simulink library "Simple_lib"  (R2018b)
settings: Solver=ode45  StartTime=0.0  StopTime=10.0  RelTol=1e-3  EnableMultiTasking=on
undefined symbols (not defined in the file or in its folder): Acceptance, beta, C, C_J, C_P, c_wall, dGain, DiscIntNeverNeededParam, Duplex, Electrical_lib, grab, h_fe, i, i3, K_T, Kman, KmanCE, mu_s, n_rev, R_arm, Simplex, systemTs, tau_0, TinIC, Ts, w_0, wallMass, Watch_lib
libraries: $bdroot x407, PlantUtilityBlockset_lib x30, peGeneralControl x22, simulink x11
(part 6 of 14)

== system Simple_lib/Electrical/BiGain ==
  w : Inport
  Bus Creator1 : BusCreator  Inputs=2
  Bus Selector : BusSelector  OutputSignals=I,C
  Ground : Ground
  Terminator : Terminator
  _in : $bdroot/Rotational/_in  Level=w  Flow=tau
  _out : Subsystem  Tag=Electrical  AncestorBlock=Simple_lib/Electronics/_out  mask{Level=V, Flow=I}
      mask prompts: Level "Level variable name:"; Flow "Flow variable name:"
      mask init:
      | init_out
      mask Display:
      | % This is a new mask on top of the base mask.
      | % Use "View base mask" link below to see the base mask.
      | % Icon for flow out
      | %% Complex icon
      | %plot([0 1 1], [0 0 0.4])
      | %plot([1 1 3], [0.6 1 1])
      | %plot([1 3 2 1 0 2], [0.6 0.6 0.4 0.6 0.4 0.4])
      | %patch([0 2 1],[0.4 0.4 0.6])
      | %plot([3 2 2], [1 1 0.6])
      | %plot([2.2 2.2], [1 0.6])
      | %plot([1.8 1.8], [1 0.6])
      | %plot([1.6 2.4], [0 0])
      | %plot([2 2], [0.1 -0.1])
      | %plot([2 2], [0.4 0.2])
      | %plot([2 2 3], [-0.2 -1 -1])
      | 
      | %color('white')
      | %plot([0 3], [2 2])
      | %plot([0 3], [-2 -2])
      | 
      | %% Bolder icon
      | plot([-1 0 1], [0 -1 0])
      | %patch([-1 1 0 -1], [1 1 2 1]*1-1)
      | patch([-1 -.2 -.2], [0 0 1])
      | patch([1 .2 .2], [0 0 1])
      | %patch( [-0.1 0.1 0.1 -0.1], [0 0 1 1], [1 1 1])
      | plot(0.2*[-1 1],-0.3*[1  1]+0*1.5)
      | plot([0 0],[-0.15 -0.45]+0*1.5)
      | 
      | 
      | color('white')
      | plot( [-1 1], [2 2])
      | plot( [-1 1], -[2 2])
  k_flow1 : Gain  Gain=k_flow
  k_pot : Gain  Gain=k_level
  V : Outport
  wires:
  _out/1(out) -> V/1
  Ground/1 -> Bus Creator1/2  "J"
  Bus Selector/2 -> Terminator/1  "<C>"
  w/1 -> _in/1
  _out/2(backs) -> Bus Selector/1
  k_pot/1 -> _out/1(in)
  Bus Creator1/1 -> _in/2
  k_flow1/1 -> Bus Creator1/1  "tau"
  _in/1 -> k_pot/1
  Bus Selector/1 -> k_flow1/1  "<I>"

== system Simple_lib/Electrical/C ==
  In1 : Inport
  Bus Creator : BusCreator  Inputs=2
  Bus Selector : BusSelector  OutputSignals=V,R
  Constant : Constant  Value=C
  Divide : Product  Inputs=/*
  Ground : Ground
  Ground1 : Ground
  Inflow : $bdroot/Utility/Inflow  SystemSampleTime=-1
  Integrator (Discrete or Continuous) : peGeneralControl/Integrator (Discrete or Continuous)  LabelModeActiveChoice=Discrete  ExternalReset=level  LimitType=Anti-windup  B=inf  A=-inf  Ts=-1
  Outflow : $bdroot/Utility/Outflow  Tag=Electrical  SystemSampleTime=-1
  Sum2 : Sum  Inputs=|+-
  Sum3 : Sum  Inputs=+  CollapseMode=Specified dimension  CollapseDim=2
  Terminator : Terminator
  Weighted Sample Time2 : SampleTimeMath  TsampMathOp=/  weightValue=1
  Out1 : Outport
  wires:
  Outflow/1 -> Out1/1
  Bus Creator/1 -> Outflow/1
  Sum2/1 -> Bus Creator/1  "V"
  Sum3/1 -> Inflow/2, Divide/2  "I"
  Bus Selector/1 -> Sum2/1  "<V>"
  Integrator (Discrete or Continuous)/1 -> Sum2/2
  Outflow/2 -> Sum3/1
  Inflow/1 -> Bus Selector/1
  In1/1 -> Inflow/1
  Bus Selector/2 -> Bus Creator/2, Weighted Sample Time2/1  "<R>"
  Ground/1 -> Integrator (Discrete or Continuous)/3
  Ground1/1 -> Integrator (Discrete or Continuous)/2
  Weighted Sample Time2/1 -> Terminator/1  "1/C"
  Divide/1 -> Integrator (Discrete or Continuous)/1
  Constant/1 -> Divide/1

== system Simple_lib/Electrical/C0 ==
  C : $bdroot/Electrical/C  C=C
      settings: AttributesFormatString=%<C> (F)
  Gnd : $bdroot/Electrical/Gnd  SystemSampleTime=-1
  Out1 : Outport
  wires:
  Gnd/1 -> C/1
  C/1 -> Out1/1

== system Simple_lib/Electrical/C1 ==
  In1 : Inport
  In2 : Inport  Port=2
  1/R1 : Gain  Gain=-1
  1/R2 : Gain  Gain=-1
  Capacitance : Gain  Gain=C
  Discrete-Time Integrator2 : DiscreteIntegrator  gainval=1  SampleTime=Ts  ICPrevOutput=DiscIntNeverNeededParam  ICPrevScaledInput=DiscIntNeverNeededParam
  Simplex : PlantUtilityBlockset_lib/Utility/Push  Tag=Electrical  SystemSampleTime=-1
  Simplex1 : PlantUtilityBlockset_lib/Utility/Push  Tag=Electrical  SystemSampleTime=-1
  Sum : Sum  Inputs=+|+
  Sum1 : Sum  Inputs=|+-
  Unit Delay : UnitDelay  SampleTime=-1
  big : Gain  Gain=100
  wires:
  big/1 -> Discrete-Time Integrator2/1, Capacitance/1
  In1/1 -> Simplex/1
  Simplex/1 -> 1/R2/1
  1/R2/1 -> Sum/1
  Sum/1 -> Sum1/1
  In2/1 -> Simplex1/1
  Simplex1/1 -> Sum/2
  1/R1/1 -> Simplex1/2
  Sum1/1 -> big/1
  Discrete-Time Integrator2/1 -> Sum1/2
  Capacitance/1 -> Unit Delay/1
  Unit Delay/1 -> Simplex/2, 1/R1/1

== system Simple_lib/Electrical/C2 ==
  In1 : Inport
  C1 : $bdroot/Electrical/C1  C=1
  Gnd : $bdroot/Electrical/Gnd  SystemSampleTime=-1
  wires:
  In1/1 -> C1/2
  Gnd/1 -> C1/1

== system Simple_lib/Electrical/Can ==
  note: {\bfCAN - arbitrates contention by {\ithats in ring} algorithm}
      |
      | The bus can arbitrate by broadcasting the minimum contender id and the sum of all contender messages.
      | This mimics the lossless bitwise arbitration method of contention resolution.
  InPot : Inport  Tag=NOFLUX
  FlowSum1 : Sum  Inputs=1  SaturateOnIntegerOverflow=on  InputSameDT=on  OutDataTypeStr=Inherit: Same as first input
  FlowSum2 : Sum  Inputs=3  SaturateOnIntegerOverflow=on  InputSameDT=on  OutDataTypeStr=Inherit: Same as first input
  MinMax : MinMax
  Mux : Mux  Inputs=3
  Mux1 : Mux  Inputs=3
  Mux2 : Mux  Inputs=3
  Selector : Selector  InputPortWidth=3  IndexOptions=Index vector (dialog)  Indices=1  OutputSizes=1
  Selector1 : Selector  InputPortWidth=3  IndexOptions=Index vector (dialog)  Indices=1  OutputSizes=1
  Selector2 : Selector  InputPortWidth=3  IndexOptions=Index vector (dialog)  Indices=1  OutputSizes=1
  Selector3 : Selector  InputPortWidth=3  IndexOptions=Index vector (dialog)  Indices=2  OutputSizes=1
  Selector5 : Selector  InputPortWidth=3  IndexOptions=Index vector (dialog)  Indices=2  OutputSizes=1
  Selector6 : Selector  InputPortWidth=3  IndexOptions=Index vector (dialog)  Indices=2  OutputSizes=1
  Selector7 : Selector  InputPortWidth=3  IndexOptions=Index vector (dialog)  Indices=3  OutputSizes=1
  Selector8 : Selector  InputPortWidth=3  IndexOptions=Index vector (dialog)  Indices=3  OutputSizes=1
  Selector9 : Selector  InputPortWidth=3  IndexOptions=Index vector (dialog)  Indices=3  OutputSizes=1
  OutPot : Outport
  OutFlow : Outport  Tag=NOFLUX  Port=2
  wires:
  InPot/1 -> OutPot/1  "p_DuplexInverter_test0"
  Mux/1 -> MinMax/1
  Mux1/1 -> OutFlow/1
  Selector5/1 -> Mux2/2
  Selector3/1 -> Mux2/1
  Selector6/1 -> Mux2/3
  Mux2/1 -> FlowSum1/1  "msg"
  MinMax/1 -> Mux1/1  "id"
  Selector/1 -> Mux/1
  Selector1/1 -> Mux/2
  Selector2/1 -> Mux/3
  Selector7/1 -> FlowSum2/1
  Selector9/1 -> FlowSum2/3
  Selector8/1 -> FlowSum2/2
  FlowSum2/1 -> Mux1/3
  FlowSum1/1 -> Mux1/2  "msg"

== system Simple_lib/Electrical/Capacitor ==
  In1 : Inport
  Discrete-Time Integrator1 : DiscreteIntegrator  gainval=1  SampleTime=-1  ICPrevOutput=DiscIntNeverNeededParam  ICPrevScaledInput=DiscIntNeverNeededParam
  Gain : Gain  Gain=-1/C
  Input : $bdroot/Utility/Input  Level=V  Flow=I
  Output : $bdroot/Utility/Output  Tag=Electrical  Level=Level  Flow=flow
  Sum : Sum  Inputs=|++
  Sum1 : Sum  Inputs=1
  Out1 : Outport
  wires:
  Discrete-Time Integrator1/1 -> Sum/2
  In1/1 -> Input/1
  Output/1 -> Out1/1
  Output/2 -> Sum1/1
  Input/1 -> Sum/1
  Sum/1 -> Output/1
  Gain/1 -> Discrete-Time Integrator1/1
  Sum1/1 -> Input/2, Gain/1

== system Simple_lib/Electrical/Complex Ammeter ==
  note: $\tau = {L \over R} > \tt{T_s}$
  note: So smaller delay comes from larger resistance
  note: It has to be able to jump through a rate change block!
  + : Inport
  - : Inport  Port=2
  1/R5 : Gain  Gain=-1
  Abs : Abs
  Abs1 : Abs
  Complex to Real-Imag : ComplexToRealImag
  Complex to Real-Imag2 : ComplexToRealImag
  Constant : Constant  Value=Ts
  Constant1 : Constant  Value=1.5
  Discrete-Time Integrator1 : DiscreteIntegrator  gainval=1  SampleTime=Ts  ICPrevOutput=DiscIntNeverNeededParam  ICPrevScaledInput=DiscIntNeverNeededParam
  Divide : Product  Inputs=***
  Divide1 : Product  Inputs=/*
  InNeg : $bdroot/Utility/Input  Level=V  Flow=I
  InPos : $bdroot/Utility/Input  Level=V  Flow=I
  Sum : Sum  Inputs=+|-
  Sum1 : Sum  Inputs=+|+
  Output : Outport
  wires:
  -/1 -> InNeg/1
  +/1 -> InPos/1
  Divide/1 -> Divide1/1  "L"
  Abs/1 -> Sum1/1
  Abs1/1 -> Sum1/2
  Constant/1 -> Divide/2
  Constant1/1 -> Divide/1
  Sum1/1 -> Divide/3
  Complex to Real-Imag/2 -> Abs/1
  Complex to Real-Imag2/2 -> Abs1/1
  Sum/1 -> Divide1/2  "DV"
  Complex to Real-Imag2/1 -> Sum/2
  Complex to Real-Imag/1 -> Sum/1
  1/R5/1 -> InNeg/2
  Discrete-Time Integrator1/1 -> 1/R5/1, Output/1, InPos/2
  InPos/1 -> Complex to Real-Imag/1
  Divide1/1 -> Discrete-Time Integrator1/1
  InNeg/1 -> Complex to Real-Imag2/1

== system Simple_lib/Electrical/Complex Resistance ==
  In1 : Inport
  Constant : Constant  Value=-1
  In : $bdroot/Utility/Input  Tag=Electrical  Level=V  Flow=I
  Out : $bdroot/Utility/Output  Tag=Electrical  Level=Level  Flow=flow
  Real-Imag to Complex : RealImagToComplex
  Sum : Sum  Inputs=|+-
  resistance : Gain  Gain=R
  Out1 : Outport
  wires:
  Out/2 -> In/2, Real-Imag to Complex/1
  Sum/1 -> Out/1
  In/1 -> Sum/1
  Out/1 -> Out1/1
  In1/1 -> In/1
  resistance/1 -> Sum/2
  Constant/1 -> Real-Imag to Complex/2
  Real-Imag to Complex/1 -> resistance/1

== system Simple_lib/Electrical/Controller ==
  InPot : Inport
  InFlow : Inport  Tag=NOFLUX  Port=2
  OutPot : Outport  Tag=NOFLUX
  tag scope: SuggestionTx1Bus_test=global
  wires:
  InPot/1 -> OutPot/1  "pot"
  InFlow/1 -> [SuggestionTx1Bus_test]  "flow"

== system Simple_lib/Electrical/D ==
  note: Put the exponential terms from Ebers Moll in here
  In1 : Inport
  In2 : Inport  Port=2
  1/R1 : Gain  Gain=-1
  1/R2 : Gain  Gain=-1
  Constant : Constant
  Input : $bdroot/Utility/Input  Level=V  Flow=I
  Input1 : $bdroot/Utility/Input  Level=V  Flow=I
  Math Function : Math  SaturateOnIntegerOverflow=on
  Sum : Sum  Inputs=+|+
  Sum1 : Sum  Inputs=|+-
  conductance : Gain  Gain=1/26e-3
  conductance1 : Gain  Gain=1e-12
  wires:
  conductance/1 -> Math Function/1
  In1/1 -> Input/1
  Input/1 -> Sum/1
  Sum/1 -> conductance/1
  In2/1 -> Input1/1
  Input1/1 -> 1/R1/1
  Sum1/1 -> conductance1/1
  conductance1/1 -> Input1/2, 1/R2/1
  Constant/1 -> Sum1/2
  Math Function/1 -> Sum1/1
  1/R2/1 -> Input/2
  1/R1/1 -> Sum/2

== system Simple_lib/Electrical/DC Motor ==
  V_1 : Inport
  V_2 : Inport  Port=2
  Discrete FIR Filter : DiscreteFir  Coefficients=ones(1,10)/10
  Discrete FIR Filter1 : DiscreteFir  Coefficients=ones(1,10)/10
  Divide : Product  Inputs=*/
  Inertia : $bdroot/Rotational/Inertia  I=J_mot
      settings: AttributesFormatString=%<I> kgm^2
  LR : $bdroot/Electronics/LR  L=1e-6  R=R_arm  Phi_0=0
      settings: AttributesFormatString=|
      | %<L> H
      | %<R> Ohm
  Lump : $bdroot/Rotational/Lump  w_0=0  max_accel=inf
      settings: AttributesFormatString=%<w_0> rad/s
  R_Cu : $bdroot/Electronics/R  Commented=on  R=R_arm
      settings: AttributesFormatString=%<R> Ohms
  R_Fe : $bdroot/Electronics/R  R=R_Fe
      settings: AttributesFormatString=%<R> Ohms
  Saturation : Saturate  UpperLimit=1  LowerLimit=0
  Sum : Sum  Inputs=-+|
  Sum2 : Sum  Inputs=|-+
  Terminator1 : Terminator
  Transducer : $bdroot/Electrical/BiGain  k_level=k_flow  k_flow=k_flow
      settings: AttributesFormatString="%<k_flow>   %<k_level>"
  ePower1 : $bdroot/Electrical/Power  SystemSampleTime=-1
  ePower2 : $bdroot/Electrical/Power  SystemSampleTime=-1
  mPower : $bdroot/Rotational/Power  SystemSampleTime=-1
  w : Outport
  wires:
  Divide/1 -> Saturation/1
  Discrete FIR Filter/1 -> Divide/1  "P_mech"
  Discrete FIR Filter1/1 -> Divide/2  "P_elec"
  Saturation/1 -> Terminator1/1  "eta"
  Sum2/1 -> Discrete FIR Filter1/1
  ePower2/2 -> Sum2/1
  V_2/1 -> ePower2/1  "V"
  ePower1/2 -> Sum2/2
  V_1/1 -> ePower1/1  "V_1"
  mPower/2 -> Discrete FIR Filter/1
  mPower/1 -> Transducer/1  "w_load"
  Transducer/1 -> Sum/1  "V"
  Sum/1 -> LR/1
  ePower2/1 -> R_Fe/2, LR/2  "V"
  ePower1/1 -> Sum/2, R_Fe/1
  Lump/1 -> w/1, mPower/1, Inertia/1

== system Simple_lib/Electrical/DI ==
  note: Put the exponential terms from Ebers Moll in here
  note: V_T
  In1 : Inport
  T : Inport  Port=2
  In2 : Inport  Port=3
  1/R1 : Gain  Gain=-1
  Constant : Constant
  Divide : Product  Inputs=*/
  Divide1 : Product  Inputs=**/
  Divide2 : Product  Inputs=*/
  Gain : Gain
  I_S : Gain  Gain=1e-12
  Math Function : Math  SaturateOnIntegerOverflow=on
  Real-Imag to Complex : RealImagToComplex
  Sum : Sum  Inputs=+|-
  Sum1 : Sum  Inputs=-+|
  _1 : $bdroot/Utility/Input  Level=V  Flow=I
  _2 : $bdroot/Utility/Input  Level=V  Flow=I
  k : Constant  Value=1.38e-23
  q : Constant  Value=1.6e-19
  I : Outport
  wires:
  Gain/1 -> Divide2/1
  k/1 -> Divide1/1
  Divide1/1 -> Divide2/2, Divide/2  "V_T"
  q/1 -> Divide1/3
  T/1 -> Divide1/2
  Divide/1 -> Math Function/1
  In1/1 -> _1/1
  _1/1 -> Sum/1
  Sum/1 -> Divide/1  "D_V"
  In2/1 -> _2/1
  Sum1/1 -> I_S/1
  Constant/1 -> Sum1/1
  Math Function/1 -> Sum1/2
  Real-Imag to Complex/1 -> _1/2, 1/R1/1
  _2/1 -> Sum/2
  I_S/1 -> Gain/1, I/1, Real-Imag to Complex/1  "I"
  Divide2/1 -> Real-Imag to Complex/2  "Cond"
  1/R1/1 -> _2/2

== system Simple_lib/Electrical/DV ==
  DV : Inport
  In : Inport  Port=2
  Duplex1 : $bdroot/Utility/Output  Tag=Electrical  Level=Level  Flow=flow
  Input1 : $bdroot/Utility/Input  Level=V  Flow=I
  Input2 : $bdroot/Utility/Input  Level=V  Flow=I
  Sum : Sum  Inputs=++|
  Sum1 : Sum  Inputs=+
  Out : Outport
  wires:
  In/1 -> Input2/1
  Duplex1/1 -> Out/1
  Duplex1/2 -> Sum1/1
  Input2/1 -> Sum/2
  Sum/1 -> Duplex1/1
  DV/1 -> Input1/1
  Sum1/1 -> Input2/2, Input1/2
  Input1/1 -> Sum/1

== system Simple_lib/Electrical/Diode ==
  V1 : Inport
  dV : Inport  Port=2
  V2 : Inport  Port=3
  1/R4 : Gain  Gain=-1
  Discrete-Time Integrator : DiscreteIntegrator  gainval=KmanBE  SampleTime=-1  LimitOutput=on  LowerSaturationLimit=0  ICPrevOutput=DiscIntNeverNeededParam  ICPrevScaledInput=DiscIntNeverNeededParam
  Input : $bdroot/Utility/Input  Level=V  Flow=I
  Input1 : $bdroot/Utility/Input  Level=V  Flow=I
  Sum : Sum  Inputs=++-
  I_12 : Outport
  wires:
  1/R4/1 -> Input1/2
  dV/1 -> Sum/2
  Input1/1 -> Sum/3
  Discrete-Time Integrator/1 -> 1/R4/1, I_12/1, Input/2
  V2/1 -> Input1/1
  Sum/1 -> Discrete-Time Integrator/1
  Input/1 -> Sum/1
  V1/1 -> Input/1

== system Simple_lib/Electrical/E1 ==
  In1 : Inport
  Bus Creator : BusCreator  Inputs=2
  Ground1 : Ground
  Out1 : Outport
  wires:
  In1/1 -> Bus Creator/1  "V"
  Ground1/1 -> Bus Creator/2  "R"
  Bus Creator/1 -> Out1/1

== system Simple_lib/Electrical/EMF ==
  In1 : Inport
  Constant : Constant  Value=Vbatt
  Input1 : $bdroot/Utility/Input  Level=V  Flow=I
  Sum : Sum  Inputs=|++
  Sum1 : Sum  Inputs=+
  _ : $bdroot/Utility/Output  Tag=Electrical  Level=Level  Flow=flow
  Out1 : Outport
  wires:
  _/1 -> Out1/1
  Input1/1 -> Sum/1
  _/2 -> Sum1/1
  Constant/1 -> Sum/2
  Sum/1 -> _/1
  In1/1 -> Input1/1
  Sum1/1 -> Input1/2

== system Simple_lib/Electrical/EMachine  ==
  note: Torque Constant = 60/2/pi/K_V
  K : Inport
  V_in : Inport  Port=2
  w_rot : Inport  Port=3
  w_stat : Inport  Port=4
  Gain : Gain  Gain=-1
  Input : $bdroot/Utility/Input  Level=V  Flow=I
  Input1 : $bdroot/Utility/Input  Level=V  Flow=I
  Input2 : $bdroot/Utility/Input  Level=V  Flow=I
  Output : $bdroot/Utility/Output  Tag=Electrical  Level=Level  Flow=flow
  Sum : Sum  Inputs=-+|
  Sum1 : Sum  Inputs=|+-
  Sum3 : Sum  Inputs=+
  Times : Product  Inputs=**
  Times2 : Product  Inputs=**
  V_out : Outport
  wires:
  Gain/1 -> Input1/2
  Times2/1 -> Input2/2, Gain/1
  Times/1 -> Sum/1
  Sum3/1 -> Times2/2, Input/2
  Input2/1 -> Sum1/1
  Input1/1 -> Sum1/2
  w_stat/1 -> Input1/1
  Sum1/1 -> Times/2
  K/1 -> Times/1, Times2/1
  Output/2 -> Sum3/1
  Output/1 -> V_out/1
  Input/1 -> Sum/2
  w_rot/1 -> Input2/1
  V_in/1 -> Input/1
  Sum/1 -> Output/1

== system Simple_lib/Electrical/Flow ==
  In1 : Inport
  1/R1 : Gain  Gain=-1
  Flow : Scope
      settings: Tag=I
  Input2 : $bdroot/Utility/Input  Level=V  Flow=I
  _ : $bdroot/Utility/Output  Tag=Electrical  Level=Level  Flow=flow
  Out1 : Outport
  wires:
  Input2/1 -> _/1
  _/2 -> Input2/2, 1/R1/1
  In1/1 -> Input2/1
  _/1 -> Out1/1
  1/R1/1 -> Flow/1

== system Simple_lib/Electrical/Forward ==
  In1 : Inport
  Discrete-Time Integrator1 : DiscreteIntegrator  gainval=1/0.01  InitialCondition=-deltaV  SampleTime=Ts  LimitOutput=on  LowerSaturationLimit=-deltaV  ICPrevOutput=DiscIntNeverNeededParam  ICPrevScaledInput=DiscIntNeverNeededParam
  Input : $bdroot/Utility/Input  Level=V  Flow=I
  Sum : Sum  Inputs=|++
  _ : $bdroot/Utility/Output  Tag=Electrical  Level=Level  Flow=flow
  Out1 : Outport
  wires:
  Discrete-Time Integrator1/1 -> Sum/2
  _/1 -> Out1/1
  Sum/1 -> _/1
  _/2 -> Discrete-Time Integrator1/1, Input/2
  Input/1 -> Sum/1
  In1/1 -> Input/1

== system Simple_lib/Electrical/Gnd ==
  Input : Inport
  Bus Creator1 : BusCreator  Inputs=2
  Ground2 : Ground
  Ground3 : Ground
  I1 : $bdroot/Electrical/I1  SystemSampleTime=-1
  Output : Outport
  wires:
  Ground2/1 -> Bus Creator1/2  "R"
  Input/1 -> I1/1
  Ground3/1 -> Bus Creator1/1  "V"
  Bus Creator1/1 -> I1/2
  I1/1 -> Output/1  "I1"

== system Simple_lib/Electrical/Grnd ==
  Constant : Constant  Value=0
  Sum : Sum  Inputs=+
  _ : $bdroot/Utility/Output  Tag=Electrical  Level=Level  Flow=flow
  Gnd : Outport
  i : Outport  Port=2
  wires:
  _/1 -> Gnd/1
  Constant/1 -> _/1
  _/2 -> Sum/1
  Sum/1 -> i/1

== system Simple_lib/Electrical/H ==
  + : Inport
  Sw : Inport  Port=2
  - : Inport  Port=3
  Input1 : $bdroot/Utility/Input  Level=V  Flow=I
  Input2 : $bdroot/Utility/Input  Level=V  Flow=I
  Multiply : Product
  Multiply1 : Product
  Sum1 : Sum  Inputs=+
  Sum2 : Sum  Inputs=+
  Switch Volts : Subsystem
  _ : $bdroot/Utility/Output  Tag=Electrical  Level=Level  Flow=flow
  _1 : $bdroot/Utility/Output  Tag=Electrical  Level=Level  Flow=flow
  u : Outport
  v : Outport  Port=2
  wires:
  Sum1/1 -> Multiply/1
  Sum2/1 -> Multiply1/2
  Switch Volts/1(uSw) -> _/1
  Switch Volts/2(vSw) -> _1/1
  Multiply1/1 -> Input2/2
  Multiply/1 -> Input1/2
  Sw/1 -> Switch Volts/2(Sw), Multiply/2, Multiply1/1
  Input1/1 -> Switch Volts/1(u)
  +/1 -> Input1/1
  _1/2 -> Sum2/1
  _/2 -> Sum1/1
  _/1 -> u/1
  _1/1 -> v/1
  Input2/1 -> Switch Volts/3(v)
  -/1 -> Input2/1

== system Simple_lib/Electrical/H Bridge ==
  + : Inport
  ctrl : Inport  Port=2
  - : Inport  Port=3
  1-D Lookup Table1 : Lookup_n-D  NumberOfTableDimensions=1  BreakpointsForDimension1=[-1 0 1]  Table=[1 0 0]  InterpMethod=Nearest  InternalRulePriority=Speed  RndMeth=Simplest  InputSameDT=on
  1-D Lookup Table2 : Lookup_n-D  NumberOfTableDimensions=1  BreakpointsForDimension1=[-1 0 1]  Table=[0 0 1]  InterpMethod=Nearest  InternalRulePriority=Speed  RndMeth=Simplest  InputSameDT=on
  1-D Lookup Table3 : Lookup_n-D  NumberOfTableDimensions=1  BreakpointsForDimension1=[-1 0 1]  Table=[1 0 0]  InterpMethod=Nearest  InternalRulePriority=Speed  RndMeth=Simplest  InputSameDT=on
  1-D Lookup Table4 : Lookup_n-D  NumberOfTableDimensions=1  BreakpointsForDimension1=[-1 0 1]  Table=[0 0 1]  InterpMethod=Nearest  InternalRulePriority=Speed  RndMeth=Simplest  InputSameDT=on
  EMF1 : $bdroot/Electrical/EMF  Vbatt=4
  EMF2 : $bdroot/Electrical/EMF  Vbatt=4
  Tran{,1..3} (4 alike) : $bdroot/Electrical/Tran  SystemSampleTime=-1
  u : Outport
  v : Outport  Port=2
  wires:
  1-D Lookup Table3/1 -> Tran2/1
  1-D Lookup Table1/1 -> Tran1/1
  1-D Lookup Table2/1 -> Tran/1
  1-D Lookup Table4/1 -> Tran3/1
  ctrl/1 -> 1-D Lookup Table1/1, 1-D Lookup Table4/1, 1-D Lookup Table2/1, 1-D Lookup Table3/1
  EMF1/1 -> v/1
  -/1 -> Tran1/2, Tran3/2
  +/1 -> Tran/2, Tran2/2
  Tran3/1 -> ?
  Tran2/1 -> EMF1/1
  EMF2/1 -> u/1
  Tran/1 -> EMF2/1
  Tran1/1 -> ?

== system Simple_lib/Electrical/I1 ==
  note: $\tau = {L \over R} > \tt{T_s}$
  note: So smaller delay comes from larger resistance
  In1 : Inport
  In2 : Inport  Port=2
  Bus Selector : BusSelector  OutputSignals=V,R
  Bus Selector1 : BusSelector  OutputSignals=R,V
  Divide : Product  Inputs=/*
  Gain : Gain  Gain=-1
  Ground : Ground
  Ground1 : Ground
  Inflow1 : $bdroot/Utility/Inflow  SystemSampleTime=-1
  Inflow2 : $bdroot/Utility/Inflow  SystemSampleTime=-1
  Integrator (Discrete or Continuous) : peGeneralControl/Integrator (Discrete or Continuous)  LabelModeActiveChoice=Discrete  ExternalReset=level  LimitType=Anti-windup  B=inf  A=-inf  Ts=-1
  Sum : Sum  Inputs=+|-
  Sum1 : Sum  Inputs=+|+
  Weighted Sample Time2 : SampleTimeMath  TsampMathOp=*  weightValue=1
  I : Outport
  wires:
  Sum1/1 -> Weighted Sample Time2/1
  Divide/1 -> Integrator (Discrete or Continuous)/1
  In2/1 -> Inflow2/1
  In1/1 -> Inflow1/1
  Sum/1 -> Divide/2
  Integrator (Discrete or Continuous)/1 -> Gain/1, I/1, Inflow1/2
  Inflow2/1 -> Bus Selector1/1
  Weighted Sample Time2/1 -> Divide/1  "L"
  Gain/1 -> Inflow2/2
  Bus Selector/2 -> Sum1/1  "<R>"
  Bus Selector/1 -> Sum/1  "<V>"
  Ground/1 -> Integrator (Discrete or Continuous)/3
  Bus Selector1/2 -> Sum/2  "<V>"
  Ground1/1 -> Integrator (Discrete or Continuous)/2
  Bus Selector1/1 -> Sum1/2  "<R>"
  Inflow1/1 -> Bus Selector/1

== system Simple_lib/Electrical/I_1 ==
  In1 : Inport
  In2 : Inport  Port=2
  Bus Selector : BusSelector  OutputSignals=V,R
  Bus Selector1 : BusSelector  OutputSignals=R,V
  Divide : Product  Inputs=/*
  Gain : Gain  Gain=-1
  Ground : Ground
  Ground1 : Ground
  Inflow1 : $bdroot/Utility/Inflow  SystemSampleTime=-1
  Inflow2 : $bdroot/Utility/Inflow  SystemSampleTime=-1
  Integrator (Discrete or Continuous) : peGeneralControl/Integrator (Discrete or Continuous)  LabelModeActiveChoice=Discrete  ExternalReset=level  LimitType=Anti-windup  B=inf  A=-inf  Ts=-1
  Sum : Sum  Inputs=+|-
  Sum1 : Sum  Inputs=+|+
  Weighted Sample Time2 : SampleTimeMath  TsampMathOp=*  weightValue=1
  I : Outport
  wires:
  Inflow1/1 -> Bus Selector/1
  Inflow2/1 -> Bus Selector1/1
  Sum/1 -> Divide/2
  Integrator (Discrete or Continuous)/1 -> Gain/1, I/1, Inflow1/2
  In1/1 -> Inflow1/1
  In2/1 -> Inflow2/1
  Ground/1 -> Integrator (Discrete or Continuous)/3
  Ground1/1 -> Integrator (Discrete or Continuous)/2
  Bus Selector/1 -> Sum/1  "<V>"
  Bus Selector1/2 -> Sum/2  "<V>"
  Bus Selector1/1 -> Sum1/2  "<R>"
  Bus Selector/2 -> Sum1/1  "<R>"
  Weighted Sample Time2/1 -> Divide/1  "L"
  Gain/1 -> Inflow2/2
  Divide/1 -> Integrator (Discrete or Continuous)/1
  Sum1/1 -> Weighted Sample Time2/1

== system Simple_lib/Electrical/I_src ==
  In1 : Inport
  In3 : Inport  Port=2
  1/R1 : Gain  Gain=-1
  1/R2 : Gain  Gain=-1
  Duplex1 : $bdroot/Utility/Output  Tag=Electrical  Level=Level  Flow=flow
  Input : $bdroot/Utility/Input  Level=V  Flow=I
  Input1 : $bdroot/Utility/Input  Level=V  Flow=I
  Sum : Sum  Inputs=+|+
  Out1 : Outport
  wires:
  1/R2/1 -> Sum/1
  1/R1/1 -> Input/2
  In1/1 -> Input/1
  Input/1 -> 1/R2/1
  Duplex1/1 -> Out1/1
  In3/1 -> Input1/1
  Input1/1 -> Sum/2
  Duplex1/2 -> 1/R1/1, Input1/2
  Sum/1 -> Duplex1/1

== system Simple_lib/Electrical/Inline Ammeter ==
  In1 : Inport
  Input2 : $bdroot/Utility/Input  Level=V  Flow=I
  Sum : Sum  Inputs=+
  _ : $bdroot/Utility/Output  Tag=Electrical  Level=Level  Flow=flow
  Out1 : Outport
  Out2 : Outport  Port=2
  wires:
  Sum/1 -> Out2/1
  In1/1 -> Input2/1
  _/1 -> Out1/1
  Input2/1 -> _/1
  _/2 -> Input2/2, Sum/1

== system Simple_lib/Electrical/Isrc ==
  In1 : Inport
  In2 : Inport  Port=2
  In3 : Inport  Port=3
  1/R1 : Gain  Gain=-1
  1/R2 : Gain  Gain=-1
  Input : $bdroot/Utility/Input  Level=V  Flow=I
  Input1 : $bdroot/Utility/Input  Level=V  Flow=I
  Sum : Sum  Inputs=+|+
  Out1 : Outport
  wires:
  In2/1 -> 1/R1/1, Input1/2
  Input1/1 -> Sum/2
  In3/1 -> Input1/1
  Sum/1 -> Out1/1
  Input/1 -> 1/R2/1
  In1/1 -> Input/1
  1/R1/1 -> Input/2
  1/R2/1 -> Sum/1

== system Simple_lib/Electrical/L ==
  In1 : Inport
  In2 : Inport  Port=2
  1/R2 : Gain  Gain=-1
  1/R3 : Gain  Gain=1/L
  1/R5 : Gain  Gain=-1
  Discrete-Time Integrator1 : DiscreteIntegrator  gainval=1  SampleTime=Ts  ICPrevOutput=DiscIntNeverNeededParam  ICPrevScaledInput=DiscIntNeverNeededParam
  Input : $bdroot/Utility/Input  Level=V  Flow=I
  Input1 : $bdroot/Utility/Input  Level=V  Flow=I
  Sum : Sum  Inputs=+|+
  i12 : Outport
  wires:
  1/R3/1 -> Input1/2, 1/R5/1
  Input1/1 -> Sum/2
  In2/1 -> Input1/1
  Sum/1 -> Discrete-Time Integrator1/1
  1/R2/1 -> Sum/1
  Input/1 -> 1/R2/1
  In1/1 -> Input/1
  Discrete-Time Integrator1/1 -> 1/R3/1
  1/R5/1 -> i12/1, Input/2

== system Simple_lib/Electrical/L_ ==
  note: $\Phi \text{ is in Weber = Volt seconds} }$
  V_in : Inport
  Phi_in : Inport  Port=2
  Derivative : Derivative
  Duplex : $bdroot/Utility/Output  Tag=Electrical  Level=Level  Flow=flow
  Inductance per turn : Gain  Gain=L_turn
  Simplex : $bdroot/Utility/Input  Tag=Electrical  Level=V  Flow=I
  Sum : Sum  Inputs=|++
  Sum1 : Sum  Inputs=++|
  Turns : Gain  Gain=N
  V_out : Outport
  Phi_out : Outport  Port=2
  wires:
  Sum/1 -> Duplex/1
  Simplex/1 -> Sum/1
  Duplex/1 -> V_out/1
  V_in/1 -> Simplex/1
  Inductance per turn/1 -> Sum1/2, Phi_out/1
  Duplex/2 -> Simplex/2, Inductance per turn/1
  Derivative/1 -> Sum/2
  Phi_in/1 -> Sum1/1
  Sum1/1 -> Turns/1
  Turns/1 -> Derivative/1

== system Simple_lib/Electrical/L__ ==
  note: $\Phi \text{ is in Weber = Volt seconds} }$
  V_in : Inport
  Derivative : Derivative
  Duplex : $bdroot/Utility/Output  Tag=Electrical  Level=Level  Flow=flow
  Inductance : Gain  Gain=L
  Simplex : $bdroot/Utility/Input  Tag=Electrical  Level=V  Flow=I
  Sum : Sum  Inputs=|++
  V_out : Outport
  wires:
  Inductance/1 -> Derivative/1
  Derivative/1 -> Sum/2
  Duplex/2 -> Simplex/2, Inductance/1
  V_in/1 -> Simplex/1
  Duplex/1 -> V_out/1
  Simplex/1 -> Sum/1
  Sum/1 -> Duplex/1

== system Simple_lib/Electrical/L_thru ==
  In1 : Inport
  Discrete-Time Integrator1 : DiscreteIntegrator  gainval=1  SampleTime=Ts  ICPrevOutput=DiscIntNeverNeededParam  ICPrevScaledInput=DiscIntNeverNeededParam
  Duplex : $bdroot/Utility/Output  Tag=Electrical  Level=Level  Flow=flow
  Inductance : Gain  Gain=L
  Simplex : $bdroot/Utility/Input  Tag=Electrical  Level=V  Flow=I
  Sum : Sum  Inputs=|++
  Sum1 : Sum  Inputs=|+-
  big : Gain  Gain=100
  Out1 : Outport
  wires:
  Sum/1 -> Duplex/1
  Sum1/1 -> big/1
  Simplex/1 -> Sum/1
  Duplex/2 -> Simplex/2, Sum1/1
  Duplex/1 -> Out1/1
  In1/1 -> Simplex/1
  big/1 -> Discrete-Time Integrator1/1, Inductance/1
  Discrete-Time Integrator1/1 -> Sum1/2
  Inductance/1 -> Sum/2

== system Simple_lib/Electrical/Li ==
  In1 : Inport
  In2 : Inport  Port=2
  1/R2 : Gain  Gain=-1
  1/R3 : Gain  Gain=1/L
  1/R5 : Gain  Gain=-1
  Constant : Constant  Value=i/1000
  Discrete-Time Integrator1 : DiscreteIntegrator  gainval=1  SampleTime=Ts  ICPrevOutput=DiscIntNeverNeededParam  ICPrevScaledInput=DiscIntNeverNeededParam
  Input : $bdroot/Utility/Input  Level=V  Flow=I
  Input1 : $bdroot/Utility/Input  Level=V  Flow=I
  Sum : Sum  Inputs=+|+
  Sum1 : Sum  Inputs=++|
  wires:
  1/R3/1 -> Input1/2, 1/R5/1
  Input1/1 -> Sum/2
  In2/1 -> Input1/1
  Sum/1 -> Discrete-Time Integrator1/1
  1/R2/1 -> Sum/1
  Input/1 -> 1/R2/1
  In1/1 -> Input/1
  Discrete-Time Integrator1/1 -> Sum1/2
  1/R5/1 -> Input/2
  Sum1/1 -> 1/R3/1
  Constant/1 -> Sum1/1

== system Simple_lib/Electrical/Li1 ==
  note: So smaller delay comes from larger resistance
  note: $\tau = {L \over R} > \tt{T_s}$
  In1 : Inport
  In2 : Inport  Port=2
  1/R5 : Gain  Gain=-1
  Abs : Abs
  Abs1 : Abs
  Complex to Real-Imag : ComplexToRealImag
  Complex to Real-Imag2 : ComplexToRealImag
  Constant : Constant  Value=Ts
  Constant1 : Constant  Value=1.01
  Discrete-Time Integrator1 : DiscreteIntegrator  gainval=1  SampleTime=Ts  ICPrevOutput=DiscIntNeverNeededParam  ICPrevScaledInput=DiscIntNeverNeededParam
  Divide : Product  Inputs=///*
  Input : $bdroot/Utility/Input  Level=V  Flow=I
  Input1 : $bdroot/Utility/Input  Level=V  Flow=I
  Max : MinMax  Function=max  Inputs=2
  Sum : Sum  Inputs=+|-
  Output : Outport
  wires:
  Input1/1 -> Complex to Real-Imag2/1
  In2/1 -> Input1/1
  Divide/1 -> Discrete-Time Integrator1/1
  Input/1 -> Complex to Real-Imag/1
  Discrete-Time Integrator1/1 -> 1/R5/1, Output/1, Input/2
  1/R5/1 -> Input1/2
  In1/1 -> Input/1
  Complex to Real-Imag/1 -> Sum/1
  Complex to Real-Imag2/1 -> Sum/2
  Sum/1 -> Divide/4
  Complex to Real-Imag2/2 -> Abs1/1
  Complex to Real-Imag/2 -> Abs/1
  Max/1 -> Divide/3
  Constant1/1 -> Divide/1
  Constant/1 -> Divide/2
  Abs1/1 -> Max/2
  Abs/1 -> Max/1

== system Simple_lib/Electrical/Magnetic Field ==
  In1 : Inport
  Duplex : $bdroot/Utility/Output  Tag=Electrical  Level=Level  Flow=flow
  Simplex : $bdroot/Utility/Input  Tag=Electrical  Level=V  Flow=I
  Sum1 : Sum  Inputs=+
  k_flow : Gain  Gain=k_flo
  k_pot : Gain  Gain=k_lev
  Out1 : Outport
  wires:
  Sum1/1 -> k_flow/1
  k_pot/1 -> Duplex/1
  k_flow/1 -> Simplex/2
  In1/1 -> Simplex/1
  Simplex/1 -> k_pot/1
  Duplex/1 -> Out1/1
  Duplex/2 -> Sum1/1

== system Simple_lib/Electrical/Meter ==
  In1 : Inport
  Complex to Real-Imag : ComplexToRealImag
  Input2 : $bdroot/Utility/Input  Level=V  Flow=I
  Sum : Sum  Inputs=+
  Terminator : Terminator
  _ : $bdroot/Utility/Output  Tag=Electrical  Level=Level  Flow=flow
  Out1 : Outport
  Out2 : Outport  Port=2
  wires:
  Sum/1 -> Complex to Real-Imag/1
  In1/1 -> Input2/1
  _/1 -> Out1/1
  _/2 -> Sum/1, Input2/2
  Input2/1 -> _/1
  Complex to Real-Imag/1 -> Out2/1
  Complex to Real-Imag/2 -> Terminator/1

== system Simple_lib/Electrical/NPN ==
  Collector : Inport
  Base : Inport  Port=2
  Emitter : Inport  Port=3
  DiodeBE : $bdroot/Electrical/SimpleDiode  K_diode=KmanBE
  DiodeCE : $bdroot/Electrical/SimpleDiode  K_diode=KmanCE
  Transistor Action : Subsystem
  wires:
  Transistor Action/1(dV_BE) -> DiodeBE/2
  Transistor Action/2(dV_CE) -> DiodeCE/2
  Collector/1 -> DiodeCE/1
  Base/1 -> DiodeBE/1
  Emitter/1 -> DiodeBE/3, DiodeCE/3

== system Simple_lib/Electrical/NPNwp ==
  Collector : Inport
  Base : Inport  Port=2
  Emitter : Inport  Port=3
  Constant : Constant  Value=-0.7
  Constant1 : Constant  Value=-0.7
  Diode : $bdroot/Electrical/Diode  SystemSampleTime=-1
  Diode1 : $bdroot/Electrical/Diode  SystemSampleTime=-1
  Isrc : $bdroot/Electrical/Isrc  SystemSampleTime=-1
  Isrc1 : $bdroot/Electrical/Isrc  SystemSampleTime=-1
  Sum : Sum  Inputs=+|-
  Terminator : Terminator
  Terminator1 : Terminator
  alpha_F : Gain  Gain=-0.98
  alpha_R : Gain  Gain=0.9
  Ic : Outport
  wires:
  Isrc/1 -> Terminator1/1
  Isrc1/1 -> Terminator/1
  Emitter/1 -> Diode1/3, Isrc1/1
  Base/1 -> Diode1/1, Diode/1, Isrc1/3, Isrc/3
  Collector/1 -> Diode/3, Isrc/1
  Diode/1 -> [I_CD], Sum/2
  [I_ED] -> alpha_F/1
  alpha_F/1 -> Sum/1, Isrc/2
  [I_CD] -> alpha_R/1
  alpha_R/1 -> Isrc1/2
  Diode1/1 -> [I_ED]
  Constant/1 -> Diode/2
  Constant1/1 -> Diode1/2
  Sum/1 -> Ic/1

== system Simple_lib/Electrical/OpAmp ==
  + : Inport
  - : Inport  Port=2
  Discrete-Time Integrator : DiscreteIntegrator  gainval=K_op  SampleTime=-1  ICPrevOutput=DiscIntNeverNeededParam  ICPrevScaledInput=DiscIntNeverNeededParam
  Sum : Sum  Inputs=+|-
  Out1 : Outport
  wires:
  +/1 -> Sum/1
  Sum/1 -> Discrete-Time Integrator/1
  -/1 -> Sum/2
  Discrete-Time Integrator/1 -> Out1/1

== system Simple_lib/Electrical/P ==
  Discrete-Time Integrator1 : DiscreteIntegrator  gainval=1  SampleTime=Ts  ICPrevOutput=DiscIntNeverNeededParam  ICPrevScaledInput=DiscIntNeverNeededParam
  Gain : Gain  Gain=-1/C_P
  Sum1 : Sum  Inputs=1
  _ : $bdroot/Utility/Output  Tag=Electrical  Level=Level  Flow=flow
  Out1 : Outport
  wires:
  _/1 -> Out1/1
  _/2 -> Sum1/1
  Discrete-Time Integrator1/1 -> Gain/1
  Sum1/1 -> Discrete-Time Integrator1/1
  Gain/1 -> _/1

== system Simple_lib/Electrical/PNPwp ==
  Collector : Inport
  Base : Inport  Port=2
  Emitter : Inport  Port=3
  Constant : Constant  Value=-0.7
  Constant1 : Constant  Value=-0.7
  Diode : $bdroot/Electrical/Diode  SystemSampleTime=-1
  Diode1 : $bdroot/Electrical/Diode  SystemSampleTime=-1
  Isrc : $bdroot/Electrical/Isrc  SystemSampleTime=-1
  Isrc1 : $bdroot/Electrical/Isrc  SystemSampleTime=-1
  Sum : Sum  Inputs=-|+
  Terminator : Terminator
  Terminator1 : Terminator
  alpha_F : Gain  Gain=-0.98
  alpha_R : Gain  Gain=0.9
  Ic : Outport
  wires:
  Base/1 -> Diode/3, Diode1/3, Isrc/1, Isrc1/1
  Isrc1/1 -> Terminator1/1
  Isrc/1 -> Terminator/1
  Emitter/1 -> Diode/1, Isrc/3
  Collector/1 -> Diode1/1, Isrc1/3
  Diode1/1 -> Sum/2, [I_CD]
  [I_ED] -> alpha_F/1
  alpha_F/1 -> Sum/1, Isrc1/2
  [I_CD] -> alpha_R/1
  alpha_R/1 -> Isrc/2
  Diode/1 -> [I_ED]
  Constant/1 -> Diode1/2
  Constant1/1 -> Diode/2
  Sum/1 -> Ic/1

== system Simple_lib/Electrical/Pi ==
  note: RC ~= Ts
      | so want C to just exceed Ts * the max conductance
  Abs : Abs
  Complex to Real-Imag : ComplexToRealImag
  Constant : Constant  Value=-Ts
  Constant1 : Constant  Value=2
  Discrete-Time Integrator1 : DiscreteIntegrator  gainval=1  SampleTime=Ts  ICPrevOutput=DiscIntNeverNeededParam  ICPrevScaledInput=DiscIntNeverNeededParam
  Display : Display
  Divide : Product  Inputs=***
  Divide1 : Product  Inputs=*/
  Min : MinMax  Function=max
  Scope : Scope
  Sum1 : Sum  Inputs=1
  _ : $bdroot/Utility/Output  Tag=Electrical  Level=Level  Flow=flow
  Out1 : Outport
  wires:
  Complex to Real-Imag/2 -> Abs/1
  Divide/1 -> Divide1/2, Display/1
  Min/1 -> Divide/1
  _/1 -> Out1/1
  _/2 -> Complex to Real-Imag/1
  Discrete-Time Integrator1/1 -> _/1
  Divide1/1 -> Discrete-Time Integrator1/1
  Complex to Real-Imag/1 -> Sum1/1
  Abs/1 -> Min/1, Scope/1
  Sum1/1 -> Divide1/1
  Constant/1 -> Divide/2
  Constant1/1 -> Divide/3

== system Simple_lib/Electrical/Pj ==
  note: RC ~= Ts
      | so want C to just exceed Ts * the max conductance
  Abs : Abs
  Complex to Real-Imag : ComplexToRealImag
  Discrete-Time Integrator1 : DiscreteIntegrator  gainval=1  SampleTime=-1  ICPrevOutput=DiscIntNeverNeededParam  ICPrevScaledInput=DiscIntNeverNeededParam
  Divide1 : Product  Inputs=*/
  Min : MinMax  Function=max
  Scope : Scope
  Sum1 : Sum  Inputs=1
  Weighted Sample Time1 : SampleTimeMath  TsampMathOp=Ts Only  weightValue=-2
  _ : $bdroot/Utility/Output  Tag=Electrical  Level=Level  Flow=flow
  Out1 : Outport
  wires:
  Sum1/1 -> Divide1/1
  Abs/1 -> Min/1
  Complex to Real-Imag/1 -> Sum1/1
  Divide1/1 -> Discrete-Time Integrator1/1
  Discrete-Time Integrator1/1 -> _/1
  _/2 -> Complex to Real-Imag/1
  _/1 -> Out1/1
  Min/1 -> Weighted Sample Time1/1  "c_p"
  Weighted Sample Time1/1 -> Divide1/2
  Complex to Real-Imag/2 -> Scope/1, Abs/1

== system Simple_lib/Electrical/Power ==
  " " : Inport
  Bus Creator1 : BusCreator  Inputs=3
  Bus Selector : BusSelector  OutputSignals=I,G,C
  Multiply : Product
  _in : $bdroot/Electronics/_in  Level=V  Flow=I
  _out : $bdroot/Electronics/_out  Tag=Electrical  Level=V  Flow=I
  " " : Outport
  > : Outport  Port=2
  wires:
  Multiply/1 -> >/1
  _out/1 -> " "/1
  " "/1 -> _in/1
  Bus Creator1/1 -> _in/2
  _in/1 -> Multiply/1, _out/1  "V"
  _out/2 -> Bus Selector/1
  Bus Selector/1 -> Bus Creator1/1, Multiply/2  "<I>"
  Bus Selector/2 -> Bus Creator1/2  "<G>"
  Bus Selector/3 -> Bus Creator1/3  "<C>"

== system Simple_lib/Electrical/Q0 ==
  Collector : Inport
  Base : Inport  Port=2
  Emitter : Inport  Port=3
  Constant : Constant  Value=-0.7  SampleTime=-1
  Diode1 : $bdroot/Electrical/Diode  SystemSampleTime=-1
  Diode2 : $bdroot/Electrical/Diode  SystemSampleTime=-1
  Gain : Gain  Gain=beta
  wires:
  Constant/1 -> Diode1/2
  Emitter/1 -> Diode2/3, Diode1/3
  Base/1 -> Diode1/1
  Collector/1 -> Diode2/1
  Diode1/1 -> Gain/1
  Gain/1 -> Diode2/2

== system Simple_lib/Electrical/QTM ==
  Collector : Inport
  Base : Inport  Port=2
  Emitter : Inport  Port=3
  Constant : Constant  Value=-0.7
  Diode1 : $bdroot/Electrical/Diode  SystemSampleTime=-1
  Diode2 : $bdroot/Electrical/Diode  SystemSampleTime=-1
  TransistorMan : Subsystem
  VR : $bdroot/Electrical/VR  SystemSampleTime=-1
  wires:
  Collector/1 -> Diode2/1
  Base/1 -> Diode1/1
  Emitter/1 -> VR/1, Diode1/3
  Diode1/1 -> TransistorMan/2(I_C)
  Diode2/1 -> TransistorMan/1(I_B)
  VR/1 -> Diode2/3
  TransistorMan/1(R) -> VR/2
  Constant/1 -> Diode1/2

== system Simple_lib/Electrical/Qem ==
  Collector : Inport
  Base : Inport  Port=2
  Emitter : Inport  Port=3
  DI : $bdroot/Electrical/DI  SystemSampleTime=-1
  DI1 : $bdroot/Electrical/DI  SystemSampleTime=-1
  Isrc : $bdroot/Electrical/Isrc  SystemSampleTime=-1
  Isrc1 : $bdroot/Electrical/Isrc  SystemSampleTime=-1
  Terminator : Terminator
  Terminator1 : Terminator
  alpha_F : Gain  Gain=0.98
  alpha_R : Gain  Gain=0.9
  wires:
  Isrc/1 -> Terminator1/1
  Isrc1/1 -> Terminator/1
  Emitter/1 -> DI/3, Isrc1/1
  Base/1 -> DI1/1, Isrc1/3, Isrc/3, DI/1
  Collector/1 -> DI1/3, Isrc/1
  DI1/1 -> [I_CD]
  [I_ED] -> alpha_F/1
  alpha_F/1 -> Isrc/2
  [I_CD] -> alpha_R/1
  alpha_R/1 -> Isrc1/2
  DI/1 -> [I_ED]

== system Simple_lib/Electrical/Qh ==
  note: https://en.wikipedia.org/wiki/Bipolar_junction_transistor
  Collector : Inport
  Base : Inport  Port=2
  Emitter : Inport  Port=3
  DV : $bdroot/Electrical/DV  SystemSampleTime=-1
  I_src : $bdroot/Electrical/I_src  SystemSampleTime=-1
  TransistorMan : $bdroot/Electrical/TM/TransistorMan  SystemSampleTime=-1
  TransistorMan1 : $bdroot/Electrical/TM/TransistorMan  SystemSampleTime=-1
  h_ie : $bdroot/Electrical/Ri  R=1000
      settings: AttributesFormatString=%<R> Ohms
  h_oe : $bdroot/Electrical/Ri  R=1e6
      settings: AttributesFormatString=%<R> Ohms
  h_params : $bdroot/Utility/BiGain  k_pot=h_re  k_flow=h_fe
  wires:
  Collector/1 -> I_src/1, h_oe/1
  Emitter/1 -> DV/1, I_src/2, h_oe/2
  Base/1 -> h_ie/1
  DV/1 -> h_ie/2
  I_src/1 -> h_params/1
  h_params/1 -> DV/2

== system Simple_lib/Electrical/R ==
  In1 : Inport
  In2 : Inport  Port=2
  1/R1 : Gain  Gain=-1
  1/R2 : Gain  Gain=-1
  Input2 : $bdroot/Utility/Input  Level=V  Flow=I
  Input3 : $bdroot/Utility/Input  Level=V  Flow=I
  Sum : Sum  Inputs=+|+
  conductance : Gain  Gain=1/R
  wires:
  In2/1 -> Input3/1
  Sum/1 -> conductance/1
  In1/1 -> Input2/1
  Input3/1 -> 1/R2/1
  Input2/1 -> Sum/1
  conductance/1 -> Input2/2, 1/R1/1
  1/R2/1 -> Sum/2
  1/R1/1 -> Input3/2

== system Simple_lib/Electrical/R1 ==
  In1 : Inport
  In2 : Inport  Port=2
  1/R1 : Gain  Gain=-1
  1/R2 : Gain  Gain=-1
  Discrete-Time Integrator1 : DiscreteIntegrator  gainval=1/10/Ts  SampleTime=Ts  ICPrevOutput=DiscIntNeverNeededParam  ICPrevScaledInput=DiscIntNeverNeededParam
  Simplex : PlantUtilityBlockset_lib/Utility/Push  Tag=Electrical  SystemSampleTime=-1
  Simplex1 : PlantUtilityBlockset_lib/Utility/Push  Tag=Electrical  SystemSampleTime=-1
  Sum : Sum  Inputs=+|+
  Sum1 : Sum  Inputs=|+-
  conductance : Gain  Gain=1/R
  wires:
  Discrete-Time Integrator1/1 -> Sum1/2, 1/R1/1, Simplex/2
  Sum1/1 -> Discrete-Time Integrator1/1
  1/R1/1 -> Simplex1/2
  Simplex1/1 -> Sum/2
  In2/1 -> Simplex1/1
  Sum/1 -> conductance/1
  1/R2/1 -> Sum/1
  Simplex/1 -> 1/R2/1
  In1/1 -> Simplex/1
  conductance/1 -> Sum1/1

== system Simple_lib/Electrical/R2 ==
  In1 : Inport
  c : Inport  Port=2
  In2 : Inport  Port=3
  1/R1 : Gain  Gain=-1
  1/R2 : Gain  Gain=-1
  Discrete-Time Integrator1 : DiscreteIntegrator  gainval=1/10/Ts  SampleTime=Ts  ICPrevOutput=DiscIntNeverNeededParam  ICPrevScaledInput=DiscIntNeverNeededParam
  Simplex : Subsystem  Tag=Electrical  AncestorBlock=PlantUtilityBlockset_lib/Utility/Push  InitFcn=initSimplex
      mask Display:
      | color('white')
      | plot([0 3], [2 2])
      | plot([0 3], [-2 -2])
      | color('black')
      | 
      | plot([0 2 2 3], [1 1 0 0])
      | plot([1 3 2 1 0 2], [0.6 0.6 0.4 0.6 0.4 0.4])
      | patch([1 3 2],[0.6 0.6 0.4],[0,0,0])
      | plot([0 1 1], [1 1 0.6])
      | plot([1 1 0], [0.4 -1 -1])
  Simplex1 : Subsystem  Tag=Electrical  AncestorBlock=PlantUtilityBlockset_lib/Utility/Push  InitFcn=initSimplex
      mask Display:
      | color('white')
      | plot([0 3], [2 2])
      | plot([0 3], [-2 -2])
      | color('black')
      | 
      | plot([0 2 2 3], [1 1 0 0])
      | plot([1 3 2 1 0 2], [0.6 0.6 0.4 0.6 0.4 0.4])
      | patch([1 3 2],[0.6 0.6 0.4],[0,0,0])
      | plot([0 1 1], [1 1 0.6])
      | plot([1 1 0], [0.4 -1 -1])
  Sum : Sum  Inputs=+|+
  Sum1 : Sum  Inputs=|+-
  conductance : Product
  wires:
  conductance/1 -> Sum1/1
  In1/1 -> Simplex/1(InPot)
  Simplex/1(OutPot) -> 1/R2/1
  1/R2/1 -> Sum/1
  Sum/1 -> conductance/2
  In2/1 -> Simplex1/1(InPot)
  Simplex1/1(OutPot) -> Sum/2
  1/R1/1 -> Simplex1/2(InFlow)
  Sum1/1 -> Discrete-Time Integrator1/1
  Discrete-Time Integrator1/1 -> Simplex/2(InFlow), 1/R1/1, Sum1/2
  c/1 -> conductance/1

== system Simple_lib/Electrical/R3 ==
  In1 : Inport
  Constant : Constant  Value=-1
  Inflow : $bdroot/Utility/Inflow  SystemSampleTime=-1
  Mux : Mux  Inputs=2
  Outflow : $bdroot/Utility/Outflow  Tag=Electrical  SystemSampleTime=-1
  R : Gain  Gain=R
  Sum : Sum  Inputs=|+-
  Sum2 : Sum  Inputs=+  CollapseMode=Specified dimension  CollapseDim=2
  Out1 : Outport
  wires:
  R/1 -> Sum/2
  Mux/1 -> R/1
  Outflow/1 -> Out1/1
  Outflow/2 -> Sum2/1
  In1/1 -> Inflow/1
  Inflow/1 -> Sum/1
  Constant/1 -> Mux/2
  Sum/1 -> Outflow/1
  Sum2/1 -> Mux/1, Inflow/2

== system Simple_lib/Electrical/RL ==
  In1 : Inport
  In2 : Inport  Port=2
  L : $bdroot/Electrical/L  L=L
  R_1 : $bdroot/Electrical/R_  R=R/2
      settings: AttributesFormatString=%<R> Ohm
  R_2 : $bdroot/Electrical/R_  R=R/2
      settings: AttributesFormatString=%<R> Ohm
  i12 : Outport
  wires:
  R_2/1 -> L/2
  R_1/1 -> L/1
  In1/1 -> R_1/1
  In2/1 -> R_2/1
  L/1 -> i12/1

== system Simple_lib/Electrical/R_1 ==
  In1 : Inport
  Bus Creator : BusCreator  Inputs=2
  Bus Selector : BusSelector  OutputSignals=V,R
  Constant : Constant  Value=R
  Inflow : $bdroot/Utility/Inflow  SystemSampleTime=-1
  Outflow : $bdroot/Utility/Outflow  Tag=Electrical  SystemSampleTime=-1
  R : Gain  Gain=R
  Sum1 : Sum  Inputs=|++
  Sum2 : Sum  Inputs=|+-
  Sum3 : Sum  Inputs=+  CollapseMode=Specified dimension  CollapseDim=2
  Out1 : Outport
  wires:
  Outflow/1 -> Out1/1
  Inflow/1 -> Bus Selector/1
  Outflow/2 -> Sum3/1
  In1/1 -> Inflow/1
  Bus Creator/1 -> Outflow/1
  Constant/1 -> Sum1/2
  R/1 -> Sum2/2
  Sum3/1 -> R/1, Inflow/2  "I"
  Bus Selector/1 -> Sum2/1  "<V>"
  Sum2/1 -> Bus Creator/1  "V"
  Sum1/1 -> Bus Creator/2  "R"
  Bus Selector/2 -> Sum1/1  "<R>"

== system Simple_lib/Electrical/Reverse ==
  Vup : Inport
  Complex to Real-Imag : ComplexToRealImag
  Discrete-Time Integrator1 : DiscreteIntegrator  gainval=1/0.01  InitialCondition=deltaV  SampleTime=Ts  LimitOutput=on  UpperSaturationLimit=deltaV  ICPrevOutput=DiscIntNeverNeededParam  ICPrevScaledInput=DiscIntNeverNeededParam
  Input : $bdroot/Utility/Input  Level=V  Flow=I
  Sum : Sum  Inputs=|++
  Terminator : Terminator
  _ : $bdroot/Utility/Output  Tag=Electrical  Level=Level  Flow=flow
  Vdn : Outport
  wires:
  Discrete-Time Integrator1/1 -> Sum/2
  _/1 -> Vdn/1
  Sum/1 -> _/1
  _/2 -> Complex to Real-Imag/1, Input/2
  Input/1 -> Sum/1
  Vup/1 -> Input/1
  Complex to Real-Imag/1 -> Discrete-Time Integrator1/1
  Complex to Real-Imag/2 -> Terminator/1

== system Simple_lib/Electrical/Rh ==
  In1 : Inport
  R : Inport  Port=2
  In2 : Inport  Port=3
  1/R2 : Gain  Gain=-1
  1/R3 : Gain  Gain=-1
  Complex to Real-Imag : ComplexToRealImag
  Constant : Constant  Value=i
  Divide : Product  Inputs=*/
  Input2 : $bdroot/Utility/Input  Level=V  Flow=I
  Input3 : $bdroot/Utility/Input  Level=V  Flow=I
  Sum : Sum  Inputs=+++
  Terminator : Terminator
  Output : Outport
  wires:
  Constant/1 -> Sum/2
  1/R3/1 -> Input3/2
  1/R2/1 -> Sum/3
  Divide/1 -> Complex to Real-Imag/1, 1/R3/1, Input2/2
  Input2/1 -> Sum/1
  Input3/1 -> 1/R2/1
  In1/1 -> Input2/1
  Sum/1 -> Divide/1
  In2/1 -> Input3/1
  Complex to Real-Imag/1 -> Output/1
  Complex to Real-Imag/2 -> Terminator/1
  R/1 -> Divide/2

== system Simple_lib/Electrical/Ri ==
  In1 : Inport
  In2 : Inport  Port=2
  1/R2 : Gain  Gain=-1
  1/R3 : Gain  Gain=-1
  Constant : Constant  Value=i
  Input2 : $bdroot/Utility/Input  Level=V  Flow=I
  Input3 : $bdroot/Utility/Input  Level=V  Flow=I
  Sum : Sum  Inputs=+++
  conductance : Gain  Gain=1/R
  Output : Outport
  wires:
  In2/1 -> Input3/1
  Sum/1 -> conductance/1
  In1/1 -> Input2/1
  Input3/1 -> 1/R2/1
  Input2/1 -> Sum/1
  conductance/1 -> Output/1, Input2/2, 1/R3/1
  1/R2/1 -> Sum/3
  1/R3/1 -> Input3/2
  Constant/1 -> Sum/2

== system Simple_lib/Electrical/Rvar ==
  In1 : Inport
  In3 : Inport  Port=2
  In2 : Inport  Port=3
  1/R2 : Gain  Gain=-1
  1/R3 : Gain  Gain=-1
  Constant : Constant  Value=i
  Divide : Product  Inputs=*/
  Input2 : $bdroot/Utility/Input  Level=V  Flow=I
  Input3 : $bdroot/Utility/Input  Level=V  Flow=I
  Sum : Sum  Inputs=+++
  wires:
  In2/1 -> Input3/1
  Sum/1 -> Divide/1
  In1/1 -> Input2/1
  Input3/1 -> 1/R2/1
  Input2/1 -> Sum/1
  Divide/1 -> Input2/2, 1/R3/1
  1/R2/1 -> Sum/3
  1/R3/1 -> Input3/2
  Constant/1 -> Sum/2
  In3/1 -> Divide/2

== system Simple_lib/Electrical/S ==
  note: Swtch
  note: So smaller delay comes from larger resistance
  note: $\tau = {L \over R} > \tt{T_s}$
  In1 : Inport
  Break : Inport  Port=2
  In2 : Inport  Port=3
  1/R5 : Gain  Gain=-1
  Abs : Abs
  Abs1 : Abs
  Complex to Real-Imag : ComplexToRealImag
  Complex to Real-Imag2 : ComplexToRealImag
  Constant : Constant  Value=Ts
  Constant1 : Constant  Value=1.01
  Discrete-Time Integrator1 : DiscreteIntegrator  gainval=1  ExternalReset=level  SampleTime=Ts  ICPrevOutput=DiscIntNeverNeededParam  ICPrevScaledInput=DiscIntNeverNeededParam
  Divide : Product  Inputs=///*
  Input : $bdroot/Utility/Input  Level=V  Flow=I
  Input1 : $bdroot/Utility/Input  Level=V  Flow=I
  Max : MinMax  Function=max  Inputs=2
  Rate Limiter : RateLimiter  RisingSlewLimit=100  FallingSlewLimit=-100  SampleTimeMode=inherited
  Sum : Sum  Inputs=+|-
  Output : Outport
  wires:
  Input1/1 -> Complex to Real-Imag2/1
  In2/1 -> Input1/1
  Divide/1 -> Discrete-Time Integrator1/1
  Input/1 -> Complex to Real-Imag/1
  Discrete-Time Integrator1/1 -> Rate Limiter/1
  1/R5/1 -> Input1/2
  In1/1 -> Input/1
  Complex to Real-Imag/1 -> Sum/1
  Complex to Real-Imag2/1 -> Sum/2
  Sum/1 -> Divide/4
  Complex to Real-Imag2/2 -> Abs1/1
  Complex to Real-Imag/2 -> Abs/1
  Max/1 -> Divide/3
  Constant1/1 -> Divide/1
  Constant/1 -> Divide/2
  Abs1/1 -> Max/2
  Abs/1 -> Max/1
  Break/1 -> Discrete-Time Integrator1/2
  Rate Limiter/1 -> Input/2, Output/1, 1/R5/1

== system Simple_lib/Electrical/SimpleDiode ==
  V1 : Inport
  dV : Inport  Port=2
  V2 : Inport  Port=3
  1/R4 : Gain  Gain=-1
  Discrete-Time Integrator : DiscreteIntegrator  gainval=K_diode  SampleTime=-1  LimitOutput=on  LowerSaturationLimit=0  ICPrevOutput=DiscIntNeverNeededParam  ICPrevScaledInput=DiscIntNeverNeededParam
  Input : $bdroot/Utility/Input  Level=V  Flow=I
  Input1 : $bdroot/Utility/Input  Level=V  Flow=I
  Input2 : $bdroot/Utility/Input  Level=V  Flow=I
  Sum : Sum  Inputs=+|-
  Sum1 : Sum  Inputs=++|
  wires:
  V1/1 -> Input/1
  Input/1 -> Sum/1
  Sum/1 -> Sum1/2
  V2/1 -> Input1/1
  Discrete-Time Integrator/1 -> Input2/2, Input/2, 1/R4/1
  Input1/1 -> Sum/2
  1/R4/1 -> Input1/2
  dV/1 -> Input2/1
  Sum1/1 -> Discrete-Time Integrator/1
  Input2/1 -> Sum1/1

== system Simple_lib/Electrical/SimplestEMachine ==
  w : Inport
  Inertia : Subsystem  AncestorBlock=PlantUtilityBlockset_lib/Driveline/InertialSink
      mask Display:
      | %color('white');
      | %plot([0 4],[1 1]);
      | %plot([0 4],[-1 -1]);
      | %color('black')
      | %plot([0 2],[0 0]);
      | plot([-1 -.9 -.5 0 .5 .9 1  .9  .5  0 -.5 -.9 -1]+3,      [ 0  .5 .9 1 .9 .5 0 -.5 -.9 -1 -.9 -.5  0]);
  Transducer : Subsystem
  V : Outport
  wires:
  Transducer/1(V) -> V/1
  w/1 -> Transducer/1(w), Inertia/1(In1)

== system Simple_lib/Electrical/Switch ==
  In1 : Inport
  In2 : Inport  Port=2
  In3 : Inport  Port=3
  1/R2 : Gain  Gain=-1
  1/R3 : Gain  Gain=-1
  Divide : Product  Inputs=*/
  Input2 : $bdroot/Utility/Input  Level=V  Flow=I
  Input3 : $bdroot/Utility/Input  Level=V  Flow=I
  Sum : Sum  Inputs=+|+
  wires:
  In3/1 -> Input3/1
  Sum/1 -> Divide/1
  In1/1 -> Input2/1
  Input3/1 -> 1/R2/1
  Input2/1 -> Sum/1
  Divide/1 -> Input2/2, 1/R3/1
  1/R2/1 -> Sum/2
  In2/1 -> Divide/2
  1/R3/1 -> Input3/2

== system Simple_lib/Electrical/TM ==
  C : Inport
  E : Inport  Port=2
  Meter : $bdroot/Electrical/Meter  SystemSampleTime=-1
  Meter1 : $bdroot/Electrical/Meter  SystemSampleTime=-1
  Reverse : Subsystem  AncestorBlock=Lumped_lib/Electrical/Reverse  mask{deltaV=0.6}
      mask prompts: deltaV "Potential Drop (V)"
      mask Display:
      | patch( [0 -0.05 -0.05 0],[-1 -1 1 1])
      | patch( [0 1 1],[0 1 -1])
  Rman : Subsystem  AncestorBlock=Lumped_lib/Electrical/Rvar
      mask Display:
      | %plot( [ -1 1 -1 1 -1 1 -1],[-3:3]/6)
      | %plot( [ .2 0 -.2],[ -0.4 -.5 -.4])
      | plot( [ 0 1 1 -1 -1 0 ],[-2 -1.33 1.33 1.33 -1.33 -2])
      | 
      | color('white')
      | plot([-1 1], [2 2])
      | %color('red')
      | %plot([-1 1], -[2 2])
  TransistorMan : Subsystem
  B : Outport
  wires:
  C/1 -> Meter/1
  Reverse/1(Vdn) -> Meter1/1
  Meter1/1 -> B/1
  E/1 -> Rman/3(In2), Reverse/1(Vup)
  TransistorMan/1(cond) -> Rman/2(In3)
  Meter/2 -> TransistorMan/1(I_C)
  Meter1/2 -> TransistorMan/2(I_B)
  Meter/1 -> Rman/1(In1)
